simulink model "cirrusSR22T_v65"  (R2023a)
settings: Solver=ode45  StartTime=0.0  StopTime=360  FixedStep=0.001  MaxStep=0.1  RelTol=1e-3  EnableMultiTasking=on
values from neighbouring files (symbols this model uses):
  Aero_RP = [-1.145  0.0 -0.53]*[-1 0 0;0 1 0;0 0 -1]    [sr22t_data.m]
  aileron_limits = [-0.35 0.35]    [sr22t_data.m]
  Bw = 25.99*0.3048    (= 7.921752)    [sr22t_data.m]
  CD_alpha = [-1.57    1.500 ... (first row only)    [sr22t_data.m]
  CD_beta = [-1.57    1.230 ... (first row only)    [sr22t_data.m]
  CD_elev = 0.01    [sr22t_data.m]
  CD_ind = 0.007    [sr22t_data.m]
  CD_mach = [0, 0 ... (first row only)    [sr22t_data.m]
  Cl_ail = 0.1    [sr22t_data.m]
  CL_alpha = [-0.20 -0.750 ... (first row only)    [sr22t_data.m]
  Cl_beta = -0.1    [sr22t_data.m]
  CL_elev = 0.15    [sr22t_data.m]
  Cl_p = -0.4    [sr22t_data.m]
  CL_q = 3.9 * 0    (= 0)    [sr22t_data.m]
  Cl_r = 0.15    [sr22t_data.m]
  Cl_rudder = 0.01    [sr22t_data.m]
  Cm_alpha = -0.8    [sr22t_data.m]
  Cm_alpha_dot = -7    [sr22t_data.m]
  Cm_elev = [0.0, -1.100 ... (first row only)    [sr22t_data.m]
  Cm_q = -15    [sr22t_data.m]
  Cn_ail = -0.01    [sr22t_data.m]
  Cn_beta = 0.12    [sr22t_data.m]
  Cn_r = -0.15    [sr22t_data.m]
  Cn_rudder = -0.15    [sr22t_data.m]
  Cw = 5.58*0.3048    (= 1.700784)    [sr22t_data.m]
  CY_beta = -1    [sr22t_data.m]
  CY_p = [0.0000  -0.075 ... (first row only)    [sr22t_data.m]
  CY_r = [0.0000   0.214 ... (first row only)    [sr22t_data.m]
  CY_rudder = 0.187    [sr22t_data.m]
  Den = tf_linsys1(3,2).Denominator{1,1}    [controller_h_hold.m]
  elevator_limits = [-0.35 0.35]    [sr22t_data.m]
  He = tf_linsys1(3,2).Numerator{1,1}    [controller_h_hold.m]
  Href = 0.05 * x0(3)    [controller_h_hold.m]
  Ht = tf_linsys1(3,4).Numerator{1,1}    [controller_h_hold.m]
  isTrimming = 0    [sr22t_data.m]
  Jxx = 897*1.3558179    (= 1216.1686563)    [sr22t_data.m]
  Jxz = 0    [sr22t_data.m]
  Jyy = 20699*1.3558179    (= 28064.0747121)    [sr22t_data.m]
  Jzz = 19876*1.3558179    (= 26948.2365804)    [sr22t_data.m]
  Kp = 6    [controller_h_hold.m]
  kp = 0.005    [controller_h_hold.m]
  Kq = 3    [controller_h_hold.m]
  M = 2348*0.45359237    (= 1065.03488476)    [sr22t_data.m]
  Qe = tf_linsys1(8,2).Numerator{1,1}    [controller_h_hold.m]
  Qt = tf_linsys1(8,4).Numerator{1,1}    [controller_h_hold.m]
  Rcg = [-1.25 0.00 -0.54]*[-1 0 0;0 1 0;0 0 -1]    [sr22t_data.m]
  Rengine = [-3.6 0.0 -0.09045]*[-1 0 0;0 1 0;0 0 -1]    [sr22t_data.m]
  rudder_limits = [-0.35 0.35]    [sr22t_data.m]
  Sw = 144.92*0.09290304    (= 13.4635085568)    [sr22t_data.m]
  tau = 30    [controller_h_hold.m]
  Thetae = tf_linsys1(11,2).Numerator{1,1}    [controller_h_hold.m]
  Thetat = tf_linsys1(11,4).Numerator{1,1}    [controller_h_hold.m]
  thrust_limits = [0 1]    [sr22t_data.m]
  Ti = 17.5    [controller_h_hold.m]
  Tmax = M*10    (= 10650.3488476)    [sr22t_data.m]
  u0 = [op_trim1.Inputs(1,1).u, op_trim1.Inputs(2,1).u, op_trim1.Inputs(3,1).u, op_trim1.Inputs(4,1).u].'    [controller_h_hold.m]    (also in sr22t_data.m = [0, -0.013822, 0, 0.11837].')
  Ue = tf_linsys1(4,2).Numerator{1,1}    [controller_h_hold.m]
  Ut = tf_linsys1(4,4).Numerator{1,1}    [controller_h_hold.m]
  We = tf_linsys1(6,2).Numerator{1,1}    [controller_h_hold.m]
  Wt = tf_linsys1(6,4).Numerator{1,1}    [controller_h_hold.m]
  x0 = zeros(12,1)    [controller_h_hold.m]    (also in sr22t_data.m)
(part 1 of 2)
settings Model: Creator=torres  LastModifiedBy=santi
settings SolverCC: AlgebraicLoopSolver=TrustRegion
settings DataIOCC: LimitDataPoints=on  SaveFormat=Array  SignalLoggingSaveFormat=ModelDataLogs  SaveOutput=off  SaveTime=off  ReturnWorkspaceOutputs=off  SignalLoggingName=sigsOut
settings OptimizationCC: InitFltsAndDblsToZero=on  LifeSpan=inf
settings DebuggingCC: SaveWithParameterizedLinksMsg=none  UnderspecifiedInitializationDetection=Classic  MergeDetectMultiDrivingBlocksExec=none  SignalResolutionControl=TryResolveAllWithWarning  MultiTaskDSMMsg=warning  MultiTaskCondExecSysMsg=none  FcnCallInpInsideContextMsg=warning  UnconnectedInputMsg=warning  UnconnectedOutputMsg=warning  UnconnectedLineMsg=warning  SFUnexpectedBacktrackingDiag=warning  SFNoUnconditionalDefaultTransitionDiag=warning  SFExecutionAtInitializationDiag=none  ArithmeticOperatorsInVariantConditions=warning
settings HardwareCC: ProdBitPerPointer=32  ProdBitPerSizeT=32  ProdBitPerPtrDiffT=32  ProdLargestAtomicFloat=None  ProdIntDivRoundTo=Undefined  ProdEndianess=Unspecified  ProdWordSize=32  ProdHWDeviceType=32-bit Generic  TargetHWDeviceType=32-bit Generic  TargetUnknown=on  ProdEqTarget=off
settings ModelReferenceCC: PropagateSignalLabelsOutOfModel=off
settings CodeAppCC: StateflowObjectComments=on
settings GRTTargetCC: TargetFcnLib=ansi_tfl_tmw.mat  TargetLangStandard=C89/C90 (ANSI)  CombineOutputUpdateFcns=off  GRTInterface=on
settings ConfigComp: CovMetricSettings=dw  CovSaveCumulativeToWorkspaceVar=on  CovSaveSingleToWorkspaceVar=on

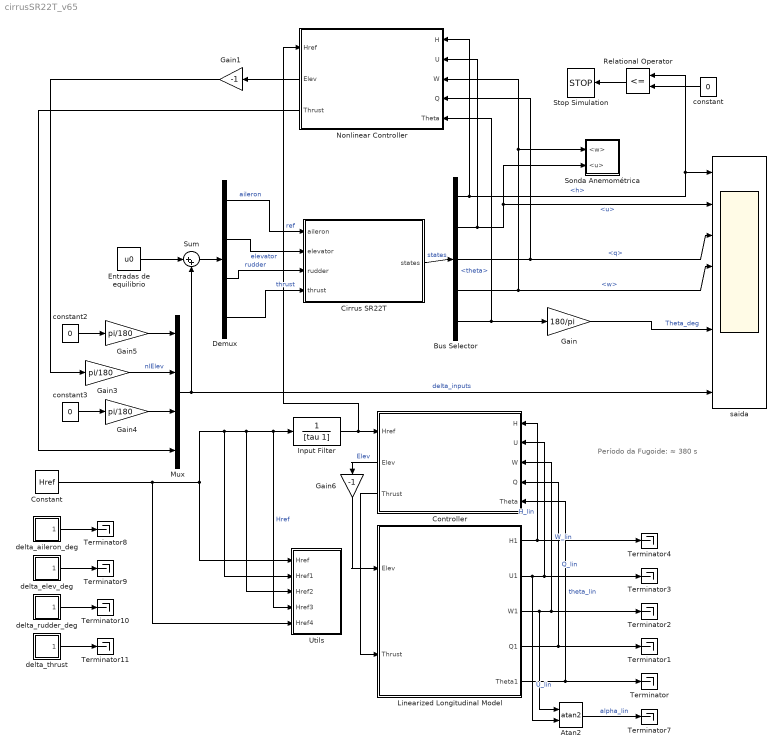
== system cirrusSR22T_v65 ==
  note: Período da Fugoide:
      | ≈ 380 s
  Atan2 : Trigonometry  Operator=atan2
  Bus Selector : BusSelector  OutputSignals=h,u,q,w,theta
  Cirrus SR22T : Subsystem
      mask Display: image(imread('SR22T.png'))
  Constant : Constant  Value=Href
  Controller : Subsystem
      settings: PortSchema="{\"entries\":[{\"content\":{\"sides\":[{\"content\":{\"connectorIds\":[\"In1\",\"In2\",\"In3\",\"In4\",\"In5\"]},\"type\":\"ConnectorPlacement.EquallySpacedRectSide\",\"uuid\":\"9a383977-e38d-4d96-a3fa-0666e6dce92b\"},{\"content\":{\"connectorIds\":[\"In6\",\"Out1\",\"Out2\"],\"side\":\"RIGHT\"},\"type\":\"ConnectorPlacement.EquallySpacedRectSide\",\"uuid\":\"65d7c93f-963c-4d71-9e25-46c931ae3c13\"},{\"content\":{\"side\":\"TOP\"},\"type\":\"ConnectorPlacement.EquallySpacedRectSide\",\"uuid\":\"543da9eb-7754-41f0-af2e-6eb03e83efa0\"}]},\"type\":\"ConnectorPlacement.EquallySpacedConnector\",\"uuid\":\"2a52e937-2907-406d-a0c6-1b75b66257ee\"}],\"packageUris\":[\"http://schema.mathworks.com/mf0/Connector/R2020b\"],\"version\":\"1.0\"}"
  Demux : Demux
      settings: DisplayOption=none
  Entradas de equilibrio : Constant  Value=u0
  Gain : Gain  Gain=180/pi  SaturateOnIntegerOverflow=on  OutDataTypeStr=Inherit: Same as input  ParamDataTypeStr=Inherit: Same as input
  Gain1 : Gain  Gain=-1
  Gain3 : Gain  Gain=pi/180  SaturateOnIntegerOverflow=on  OutDataTypeStr=Inherit: Same as input  ParamDataTypeStr=Inherit: Same as input
  Gain4 : Gain  Gain=pi/180  SaturateOnIntegerOverflow=on  OutDataTypeStr=Inherit: Same as input  ParamDataTypeStr=Inherit: Same as input
  Gain5 : Gain  Gain=pi/180  SaturateOnIntegerOverflow=on  OutDataTypeStr=Inherit: Same as input  ParamDataTypeStr=Inherit: Same as input
  Gain6 : Gain  Gain=-1
  Input Filter : TransferFcn  Denominator=[tau 1]
  Linearized Longitudinal Model : Subsystem
  Mux : Mux
  Nonlinear Controller : Subsystem
      settings: PortSchema="{\"entries\":[{\"content\":{\"sides\":[{\"content\":{\"connectorIds\":[\"In1\",\"In2\",\"In3\",\"In4\",\"In5\"]},\"type\":\"ConnectorPlacement.EquallySpacedRectSide\",\"uuid\":\"9a383977-e38d-4d96-a3fa-0666e6dce92b\"},{\"content\":{\"connectorIds\":[\"In6\",\"Out1\",\"Out2\"],\"side\":\"RIGHT\"},\"type\":\"ConnectorPlacement.EquallySpacedRectSide\",\"uuid\":\"65d7c93f-963c-4d71-9e25-46c931ae3c13\"},{\"content\":{\"side\":\"TOP\"},\"type\":\"ConnectorPlacement.EquallySpacedRectSide\",\"uuid\":\"543da9eb-7754-41f0-af2e-6eb03e83efa0\"}]},\"type\":\"ConnectorPlacement.EquallySpacedConnector\",\"uuid\":\"2a52e937-2907-406d-a0c6-1b75b66257ee\"}],\"packageUris\":[\"http://schema.mathworks.com/mf0/Connector/R2020b\"],\"version\":\"1.0\"}"
  Relational Operator : RelationalOperator  Operator=<=  InputSameDT=off
  Sonda Anemométrica : Subsystem
  Stop Simulation : Stop
  Sum : Sum  Inputs=|++  SaturateOnIntegerOverflow=on
  Terminator{,1..4,7..11} (10 alike) : Terminator
  Utils : Subsystem
  constant : Constant  Value=0
  constant2 : Constant  Value=0
  constant3 : Constant  Value=0
  delta_aileron_deg : Subsystem  mask{t0=90, dt=5, A=0}
      mask prompts: t0 "Start time"; dt "Pulse Width"; A "Amplitude"
      mask help: Doublet input to control surface.
      mask Display: plot(0,0,100,100,[90,70,70,50,50,30,30,10],[50,50,10,10,90,90,50,50])
  delta_elev_deg : Subsystem  mask{t0=20, dt=1, A=1}
      mask prompts: t0 "Start time"; dt "Pulse Width"; A "Amplitude"
      mask help: Doublet input to control surface.
      mask Display: plot(0,0,100,100,[90,70,70,50,50,30,30,10],[50,50,10,10,90,90,50,50])
  delta_rudder_deg : Subsystem  mask{t0=90, dt=1, A=0}
      mask prompts: t0 "Start time"; dt "Pulse Width"; A "Amplitude"
      mask help: Doublet input to control surface.
      mask Display: plot(0,0,100,100,[90,70,70,50,50,30,30,10],[50,50,10,10,90,90,50,50])
  delta_thrust : Subsystem  mask{t0=60, dt=1000, A=0}
      mask prompts: t0 "Start time"; dt "Duration"; A "Amplitude"
      mask Display: plot(0,0,100,100,[98,50,50,30,30,2],[20,20,80,80,20,20])
  saida : Scope  NumInputPorts=8
  wires:
  Cirrus SR22T/1(states) -> Bus Selector/1  "states"
  Bus Selector/2 -> Nonlinear Controller/2(U), saida/2, Sonda Anemométrica/2(<u>)  "<u>"
  Bus Selector/3 -> Nonlinear Controller/4(Q), saida/3  "<q>"
  Bus Selector/4 -> Nonlinear Controller/3(W), Sonda Anemométrica/1(<w>), saida/4  "<w>"
  Bus Selector/5 -> Gain/1, Nonlinear Controller/5(Theta)  "<theta>"
  Demux/1 -> Cirrus SR22T/1(aileron)  "aileron"
  Gain/1 -> saida/6  "Theta_deg"
  Demux/2 -> Cirrus SR22T/2(elevator)  "elevator"
  Demux/3 -> Cirrus SR22T/3(rudder)  "rudder"
  Demux/4 -> Cirrus SR22T/4(thrust)  "thrust"
  Entradas de equilibrio/1 -> Sum/1
  Sum/1 -> Demux/1
  constant2/1 -> Gain5/1
  Nonlinear Controller/1(Elev) -> Gain1/1
  constant3/1 -> Gain4/1
  Nonlinear Controller/2(Thrust) -> Mux/4
  Mux/1 -> Sum/2, saida/8  "delta_inputs"
  Gain3/1 -> Mux/2  "nlElev"
  Gain4/1 -> Mux/3
  Gain5/1 -> Mux/1
  Relational Operator/1 -> Stop Simulation/1
  constant/1 -> Relational Operator/2
  Bus Selector/1 -> Nonlinear Controller/1(H), Relational Operator/1, saida/1  "<h>"
  Linearized Longitudinal Model/5(Theta1) -> Controller/5(Theta), Terminator/1  "theta_lin"
  Linearized Longitudinal Model/4(Q1) -> Controller/4(Q), Terminator1/1  "Q_lin"
  Linearized Longitudinal Model/3(W1) -> Terminator2/1, Controller/3(W), Atan2/1  "W_lin"
  Linearized Longitudinal Model/2(U1) -> Terminator3/1, Controller/2(U), Atan2/2  "U_lin"
  Linearized Longitudinal Model/1(H1) -> Controller/1(H), Terminator4/1  "H_lin"
  Controller/2(Thrust) -> Linearized Longitudinal Model/2(Thrust)
  Controller/1(Elev) -> Gain6/1  "Elev"
  Gain6/1 -> Linearized Longitudinal Model/1(Elev)
  Atan2/1 -> Terminator7/1  "alpha_lin"
  delta_rudder_deg/1(Out1) -> Terminator10/1
  delta_elev_deg/1(Out1) -> Terminator9/1
  delta_aileron_deg/1(Out1) -> Terminator8/1
  delta_thrust/1(Out1) -> Terminator11/1
  Gain1/1 -> Gain3/1
  Constant/1 -> Utils/5(Href4), Utils/2(Href1), Utils/3(Href2), Utils/4(Href3), Input Filter/1, Utils/1(Href)  "Href"
  Input Filter/1 -> Nonlinear Controller/6(Href), Controller/6(Href)  "ref"

== system cirrusSR22T_v65/Cirrus SR22T ==
  note: Modelo Dinamico de Corpo Rigido
  aileron : Inport
  elevator : Inport  Port=2
  rudder : Inport  Port=3
  thrust : Inport  Port=4
  Aerodinamica : Subsystem  mask{flap=0, bw=Bw, cw=Cw, Sw=Sw}
      mask prompts: flap "Comando Flap (0, 1, 2 ou 3)"; bw "Comprimento da asa  - wingspan (m)"; cw "Corda media da asa (m)"; Sw "Area da asa (m2)"
  Atmosfera Padrao : Subsystem
  Bus Creator : BusCreator  Inputs=4
  Equations of Motion : Subsystem  mask{R_engine=Rengine, Rcg=Rcg, Aero_RP=Aero_RP, m=M, Jxz=Jxz, Jxx=Jxx, Jyy=Jyy, Jzz=Jzz, d=[0; 0; 0]}
      mask prompts: R_engine "Engine position (row vector in meters)"; Rcg "C.G. position (m)"; Aero_RP "Nominal C.G. (m) = Aerodynamic Reference Point"; m "Aircraft mass (Kg)"; Jxz "Inertia product (Jxz)"; Jxx "Inertia (Jxx)"; Jyy "Inertia (Jyy)"; Jzz "Inertia (Jzz)"; d "Accelerometers displacement from CG (vector in the ABC frame, in (m))"
  Gravidade : Constant  Value=9.807
  Propulsao : Subsystem  mask{Tmax=Tmax}
      mask prompts: Tmax "Tracao Maxima (N)"
  Saturation : Saturate  UpperLimit=aileron_limits(2)  LowerLimit=aileron_limits(1)
  Saturation1 : Saturate  UpperLimit=elevator_limits(2)  LowerLimit=elevator_limits(1)
  Saturation2 : Saturate  UpperLimit=rudder_limits(2)  LowerLimit=rudder_limits(1)
  Saturation3 : Saturate  UpperLimit=thrust_limits(2)  LowerLimit=thrust_limits(1)
  Terminator : Terminator
  Terminator1 : Terminator
  Terminator2 : Terminator
  states : Outport
  wires:
  Atmosfera Padrao/1(Atmosphere) -> Aerodinamica/3(Atmosphere)
  Equations of Motion/1(states) -> states/1, Aerodinamica/1(states), Atmosfera Padrao/1(states)
  aileron/1 -> Saturation/1  "aileron"
  elevator/1 -> Saturation1/1  "elevator"
  rudder/1 -> Saturation2/1  "rudder"
  Gravidade/1 -> Atmosfera Padrao/2(gravity), Equations of Motion/3(gravity)
  thrust/1 -> Saturation3/1  "thrust"
  Bus Creator/1 -> Aerodinamica/2(controls), Propulsao/1(controls)
  Aerodinamica/1(Faero) -> Equations of Motion/1(Faero)
  Aerodinamica/2(Maero) -> Equations of Motion/2(Maero)
  Propulsao/1(Thrust) -> Equations of Motion/4(Thrust)
  Saturation/1 -> Bus Creator/1  "aileron"
  Saturation1/1 -> Bus Creator/2  "elevator"
  Saturation2/1 -> Bus Creator/3  "rudder"
  Saturation3/1 -> Bus Creator/4  "thrust"
  Equations of Motion/2(ideal_gyro) -> Terminator/1
  Equations of Motion/4(ideal_attitude) -> Terminator2/1
  Equations of Motion/3(ideal_accelerometer) -> Terminator1/1

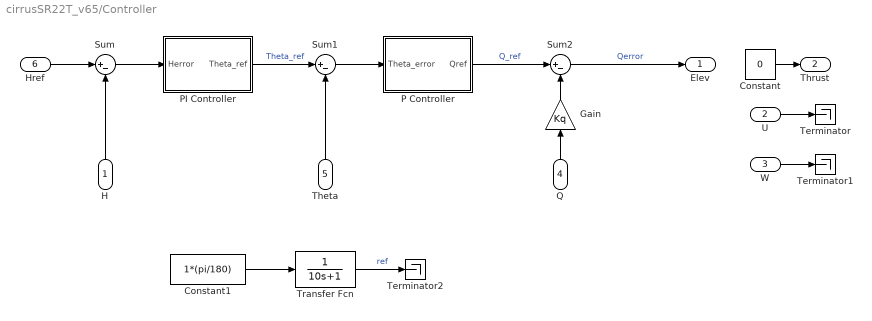
== system cirrusSR22T_v65/Controller ==
  H : Inport
  U : Inport  Port=2
  W : Inport  Port=3
  Q : Inport  Port=4
  Theta : Inport  Port=5
  Href : Inport  Port=6
  Constant : Constant  Value=0
  Constant1 : Constant  Value=1*(pi/180)  VectorParams1D=off
  Gain : Gain  Gain=Kq
  P Controller : Subsystem
  PI Controller : Subsystem
  Sum : Sum  Inputs=|+-
  Sum1 : Sum  Inputs=|+-
  Sum2 : Sum  Inputs=|+-
  Terminator : Terminator
  Terminator1 : Terminator
  Terminator2 : Terminator
  Transfer Fcn : TransferFcn  Denominator=[10 1]
  Elev : Outport
  Thrust : Outport  Port=2
  wires:
  Href/1 -> Sum/1
  Sum/1 -> PI Controller/1(Herror)
  Sum1/1 -> P Controller/1(Theta_error)
  Sum2/1 -> Elev/1  "Qerror"
  U/1 -> Terminator/1
  W/1 -> Terminator1/1
  Constant/1 -> Thrust/1
  H/1 -> Sum/2
  Theta/1 -> Sum1/2
  Q/1 -> Gain/1
  Gain/1 -> Sum2/2
  P Controller/1(Qref) -> Sum2/1  "Q_ref"
  Transfer Fcn/1 -> Terminator2/1  "ref"
  Constant1/1 -> Transfer Fcn/1
  PI Controller/1(Theta_ref) -> Sum1/1  "Theta_ref"

== system cirrusSR22T_v65/Linearized Longitudinal Model ==
  Elev : Inport
  Thrust : Inport  Port=2
  H : Subsystem
  Q : Subsystem
  Theta : Subsystem
  U : Subsystem
  W : Subsystem
  H1 : Outport
  U1 : Outport  Port=2
  W1 : Outport  Port=3
  Q1 : Outport  Port=4
  Theta1 : Outport  Port=5
  wires:
  U/1(U) -> U1/1
  Q/1(Q) -> Q1/1
  Elev/1 -> Theta/1(Elev), Q/1(Elev), W/1(Elev), U/1(Elev), H/1(Elev)
  H/1(H) -> H1/1
  Theta/1(Theta) -> Theta1/1
  Thrust/1 -> Q/2(Thrust), Theta/2(Thrust), W/2(Thrust), U/2(Thrust), H/2(Thrust)
  W/1(W) -> W1/1

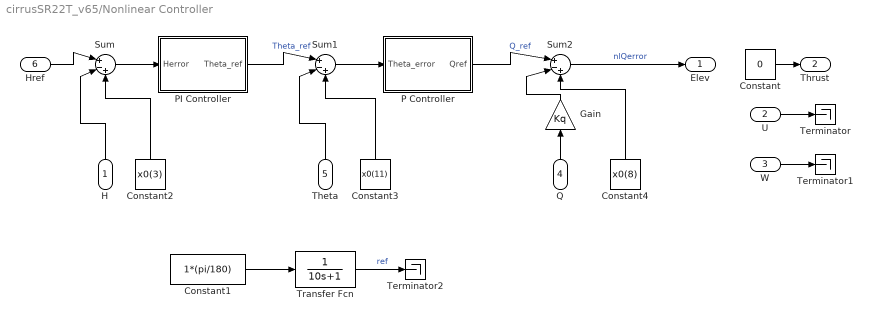
== system cirrusSR22T_v65/Nonlinear Controller ==
  H : Inport
  U : Inport  Port=2
  W : Inport  Port=3
  Q : Inport  Port=4
  Theta : Inport  Port=5
  Href : Inport  Port=6
  Constant : Constant  Value=0
  Constant1 : Constant  Value=1*(pi/180)  VectorParams1D=off
  Constant2 : Constant  Value=x0(3)
  Constant3 : Constant  Value=x0(11)
  Constant4 : Constant  Value=x0(8)
  Gain : Gain  Gain=Kq
  P Controller : Subsystem
  PI Controller : Subsystem
  Sum : Sum  Inputs=|+-+
  Sum1 : Sum  Inputs=|+-+
  Sum2 : Sum  Inputs=|+-+
  Terminator : Terminator
  Terminator1 : Terminator
  Terminator2 : Terminator
  Transfer Fcn : TransferFcn  Denominator=[10 1]
  Elev : Outport
  Thrust : Outport  Port=2
  wires:
  Href/1 -> Sum/1
  Sum/1 -> PI Controller/1(Herror)
  Sum1/1 -> P Controller/1(Theta_error)
  Sum2/1 -> Elev/1  "nlQerror"
  U/1 -> Terminator/1
  W/1 -> Terminator1/1
  Constant/1 -> Thrust/1
  H/1 -> Sum/2
  Theta/1 -> Sum1/2
  Q/1 -> Gain/1
  Gain/1 -> Sum2/2
  P Controller/1(Qref) -> Sum2/1  "Q_ref"
  Transfer Fcn/1 -> Terminator2/1  "ref"
  Constant1/1 -> Transfer Fcn/1
  PI Controller/1(Theta_ref) -> Sum1/1  "Theta_ref"
  Constant2/1 -> Sum/3
  Constant3/1 -> Sum1/3
  Constant4/1 -> Sum2/3

== system cirrusSR22T_v65/Sonda Anemométrica ==
  <w> : Inport
  <u> : Inport  Port=2
  Bus Selector3 : BusSelector  OutputSignals=VT,alpha,beta
  Gain7 : Gain  Gain=180/pi  SaturateOnIntegerOverflow=on  OutDataTypeStr=Inherit: Same as input  ParamDataTypeStr=Inherit: Same as input
  Gain8 : Gain  Gain=180/pi  SaturateOnIntegerOverflow=on  OutDataTypeStr=Inherit: Same as input  ParamDataTypeStr=Inherit: Same as input
  Mux1 : Mux  Inputs=3
  Sonda__anemometrica : Scope  NumInputPorts=3
  constant1 : Constant  Value=0
  "u,v,w -> Vt,alpha,beta" : Subsystem
  wires:
  Bus Selector3/1 -> Sonda__anemometrica/1  "<VT>"
  Gain7/1 -> Sonda__anemometrica/2  "alfa_deg"
  "u,v,w -> Vt,alpha,beta"/1(vel_wind) -> Bus Selector3/1
  Mux1/1 -> "u,v,w -> Vt,alpha,beta"/1(vel_body)
  constant1/1 -> Mux1/2
  Bus Selector3/3 -> Gain8/1  "<beta>"
  Gain8/1 -> Sonda__anemometrica/3  "beta_deg"
  Bus Selector3/2 -> Gain7/1  "<alpha>"
  <w>/1 -> Mux1/3
  <u>/1 -> Mux1/1

== system cirrusSR22T_v65/Utils ==
  Href : Inport
  Href1 : Inport  Port=2
  Href2 : Inport  Port=3
  Href3 : Inport  Port=4
  Href4 : Inport  Port=5
  Constant1 : Constant  Value=x0(3)
  Gain10 : Gain  Gain=-0.02
  Gain9 : Gain  Gain=0.02
  Sum{1..5} (5 alike) : Sum  Inputs=|++
  Terminator12 : Terminator
  Terminator5 : Terminator
  Terminator6 : Terminator
  wires:
  Sum3/1 -> Terminator5/1  "nlHref+"
  Sum5/1 -> Terminator12/1  "nlHref"
  Gain10/1 -> Sum2/1
  Href/1 -> Gain9/1
  Constant1/1 -> Sum3/2, Sum5/2, Sum4/2
  Sum4/1 -> Terminator6/1  "nlHref-"
  Sum1/1 -> Sum3/1  "Href+"
  Gain9/1 -> Sum1/1
  Sum2/1 -> Sum4/1  "Href-"
  Href4/1 -> Sum5/1
  Href1/1 -> Sum1/2
  Href3/1 -> Sum2/2
  Href2/1 -> Gain10/1

== system cirrusSR22T_v65/delta_aileron_deg ==
  Step : Step  Time=t0  After=A  SampleTime=0
  Step1 : Step  Time=t0+dt  After=-2*A  SampleTime=0
  Step2 : Step  Time=t0+2*dt  After=A  SampleTime=0
  Sum : Sum  Inputs=|++  SaturateOnIntegerOverflow=on
  Sum1 : Sum  Inputs=|++  SaturateOnIntegerOverflow=on
  Out1 : Outport
  wires:
  Step/1 -> Sum/1
  Step1/1 -> Sum/2
  Sum/1 -> Sum1/1
  Sum1/1 -> Out1/1
  Step2/1 -> Sum1/2

== system cirrusSR22T_v65/delta_elev_deg ==
  Step : Step  Time=t0  After=A  SampleTime=0
  Step1 : Step  Time=t0+dt  After=-2*A  SampleTime=0
  Step2 : Step  Time=t0+2*dt  After=A  SampleTime=0
  Sum : Sum  Inputs=|++  SaturateOnIntegerOverflow=on
  Sum1 : Sum  Inputs=|++  SaturateOnIntegerOverflow=on
  Out1 : Outport
  wires:
  Step/1 -> Sum/1
  Step1/1 -> Sum/2
  Sum/1 -> Sum1/1
  Sum1/1 -> Out1/1
  Step2/1 -> Sum1/2

== system cirrusSR22T_v65/delta_rudder_deg ==
  Step : Step  Time=t0  After=A  SampleTime=0
  Step1 : Step  Time=t0+dt  After=-2*A  SampleTime=0
  Step2 : Step  Time=t0+2*dt  After=A  SampleTime=0
  Sum : Sum  Inputs=|++  SaturateOnIntegerOverflow=on
  Sum1 : Sum  Inputs=|++  SaturateOnIntegerOverflow=on
  Out1 : Outport
  wires:
  Step/1 -> Sum/1
  Step1/1 -> Sum/2
  Sum/1 -> Sum1/1
  Sum1/1 -> Out1/1
  Step2/1 -> Sum1/2

== system cirrusSR22T_v65/delta_thrust ==
  Step : Step  Time=t0  After=A  SampleTime=0
  Step1 : Step  Time=t0+dt  After=-A  SampleTime=0
  Sum : Sum  Inputs=|++  SaturateOnIntegerOverflow=on
  Out1 : Outport
  wires:
  Sum/1 -> Out1/1
  Step/1 -> Sum/1
  Step1/1 -> Sum/2

== system cirrusSR22T_v65/Cirrus SR22T/Aerodinamica ==
  states : Inport
  controls : Inport  Port=2
  Atmosphere : Inport  Port=3
  Bus Selector : BusSelector  OutputSignals=u,v,w,p,q,r
  Bus Selector2 : BusSelector  OutputSignals=aileron,elevator,rudder
  Bus Selector3 : BusSelector  OutputSignals=VT,alpha,beta
  Bus Selector4 : BusSelector  OutputSignals=VT,alpha,beta
  Calc_qbar_Mach : Subsystem
  Derivative : Derivative
  Forcas Aerodinamicas : Subsystem
  ForcasMomentos : Scope  NumInputPorts=2
  Momentos Aerodinamicos : Subsystem
  Mux : Mux  Inputs=3
  Wind->ABC : Subsystem
  "u,v,w -> Vt,alpha,beta" : Subsystem
  Faero : Outport
  Maero : Outport  Port=2
  wires:
  Bus Selector/4 -> Forcas Aerodinamicas/4(p), Momentos Aerodinamicos/5(p)  "<p>"
  Bus Selector2/2 -> Momentos Aerodinamicos/9(elevator), Forcas Aerodinamicas/8(elevator)  "<elevator>"
  Bus Selector/6 -> Forcas Aerodinamicas/6(r), Momentos Aerodinamicos/7(r)  "<r>"
  Bus Selector4/2 -> Momentos Aerodinamicos/2(alpha), Derivative/1  "<alpha>"
  Bus Selector3/2 -> Wind->ABC/1(alpha), Forcas Aerodinamicas/2(alpha)  "<alpha>"
  Bus Selector3/3 -> Wind->ABC/2(beta), Forcas Aerodinamicas/3(beta)  "<beta>"
  Bus Selector2/1 -> Momentos Aerodinamicos/10(aileron)  "<aileron>"
  controls/1 -> Bus Selector2/1
  Bus Selector3/1 -> Forcas Aerodinamicas/1(VT), Calc_qbar_Mach/2(<VT>)  "<VT>"
  Bus Selector4/3 -> Momentos Aerodinamicos/4(beta)  "<beta>"
  Atmosphere/1 -> Calc_qbar_Mach/1(In1)
  "u,v,w -> Vt,alpha,beta"/1(vel_wind) -> Bus Selector4/1, Bus Selector3/1
  states/1 -> Bus Selector/1
  Mux/1 -> "u,v,w -> Vt,alpha,beta"/1(vel_body)
  Forcas Aerodinamicas/1(Faero_wind) -> Wind->ABC/3(V_Wind), ForcasMomentos/1
  Bus Selector2/3 -> Momentos Aerodinamicos/8(rudder), Forcas Aerodinamicas/7(rudder)  "<rudder>"
  Bus Selector4/1 -> Momentos Aerodinamicos/1(VT)  "<VT>"
  Wind->ABC/1(V_ABC) -> Faero/1
  Bus Selector/1 -> Mux/1  "<u>"
  Calc_qbar_Mach/1(qbar) -> Momentos Aerodinamicos/11(pressao_dinamica_total), Momentos Aerodinamicos/12(pressao_dinamica), Forcas Aerodinamicas/9(pressao_dinamica)
  Bus Selector/3 -> Mux/3  "<w>"
  Derivative/1 -> Momentos Aerodinamicos/3(alpha_dot)
  Bus Selector/5 -> Forcas Aerodinamicas/5(q), Momentos Aerodinamicos/6(q)  "<q>"
  Calc_qbar_Mach/2(Mach) -> Forcas Aerodinamicas/10(Mach), Momentos Aerodinamicos/13(Mach)
  Bus Selector/2 -> Mux/2  "<v>"
  Momentos Aerodinamicos/1(Maero_body) -> ForcasMomentos/2, Maero/1

== system cirrusSR22T_v65/Cirrus SR22T/Atmosfera Padrao ==
  states : Inport
  gravity : Inport  Port=2
  Bus Creator : BusCreator  Inputs=4
  Bus Selector : BusSelector  OutputSignals=h
  Calc. Densidade : Fcn  Expr=1.225*(u(1)/288.15)^(-u(2)/(-0.0065*287.04)-1)
  Calc. Pressao : Fcn  Expr=101325*(u(1)/288.15)^(-u(2)/(-0.0065*287.04))
  Calc. Temperatura : Fcn  Expr=288.15 -0.0065*u(1)
  Calc. Vel. Som : Fcn  Expr=sqrt(u*1.4*287.04)
  Mux : Mux  Inputs=2
  Mux1 : Mux  Inputs=2
  Atmosphere : Outport
  wires:
  states/1 -> Bus Selector/1
  Bus Selector/1 -> Mux/1  "<h>"
  gravity/1 -> Mux/2, Mux1/2
  Mux/1 -> Calc. Temperatura/1
  Mux1/1 -> Calc. Pressao/1, Calc. Densidade/1
  Calc. Temperatura/1 -> Mux1/1, Calc. Vel. Som/1, Bus Creator/3  "Temperatura (K)"
  Calc. Pressao/1 -> Bus Creator/4  "Pressao (Pa)"
  Calc. Densidade/1 -> Bus Creator/1  "densidade (Kg/m3)"
  Calc. Vel. Som/1 -> Bus Creator/2  "Vel_som (m/s)"
  Bus Creator/1 -> Atmosphere/1

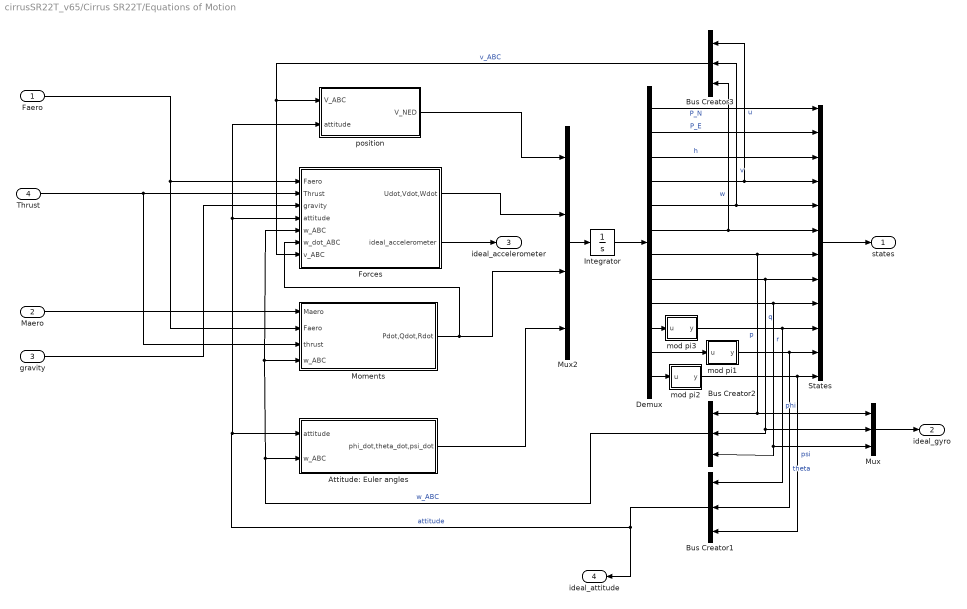
== system cirrusSR22T_v65/Cirrus SR22T/Equations of Motion ==
  Faero : Inport
  Maero : Inport  Port=2
  gravity : Inport  Port=3
  Thrust : Inport  Port=4
  Attitude: Euler angles : Subsystem
  Bus Creator1 : BusCreator  Inputs=3
  Bus Creator2 : BusCreator  Inputs=3
  Bus Creator3 : BusCreator  Inputs=3
  Demux : Demux  Outputs=12
      settings: DisplayOption=none
  Forces : Subsystem
  Integrator : Integrator  InitialCondition=x0
  Moments : Subsystem
  Mux : Mux  Inputs=3
  Mux2 : Mux
  States : BusCreator  Inputs=12
  mod pi1 : Subsystem
  mod pi2 : Subsystem
  mod pi3 : Subsystem
  position : Subsystem
  states : Outport
  ideal_gyro : Outport  Port=2
  ideal_accelerometer : Outport  Port=3
  ideal_attitude : Outport  Port=4
  wires:
  Demux/3 -> States/3  "h"
  Demux/4 -> States/4, Bus Creator3/1  "u"
  Demux/5 -> States/5, Bus Creator3/2  "v"
  Demux/6 -> States/6, Bus Creator3/3  "w"
  Demux/7 -> States/7, Bus Creator2/1, Mux/1  "p"
  Demux/8 -> States/8, Bus Creator2/2, Mux/2  "q"
  Demux/9 -> States/9, Bus Creator2/3, Mux/3  "r"
  Demux/10 -> mod pi3/1(u)
  Demux/11 -> mod pi1/1(u)
  Demux/12 -> mod pi2/1(u)
  Integrator/1 -> Demux/1
  States/1 -> states/1
  Mux2/1 -> Integrator/1
  Thrust/1 -> Moments/3(thrust), Forces/2(Thrust)
  Bus Creator1/1 -> Attitude: Euler angles/1(attitude), Forces/4(attitude), position/2(attitude), ideal_attitude/1  "attitude"
  Forces/1(Udot,Vdot,Wdot) -> Mux2/2
  gravity/1 -> Forces/3(gravity)
  Attitude: Euler angles/1(phi_dot,theta_dot,psi_dot) -> Mux2/4
  Maero/1 -> Moments/1(Maero)
  Bus Creator3/1 -> Forces/7(v_ABC), position/1(V_ABC)  "v_ABC"
  Faero/1 -> Forces/1(Faero), Moments/2(Faero)
  Bus Creator2/1 -> Attitude: Euler angles/2(w_ABC), Forces/5(w_ABC), Moments/4(w_ABC)  "w_ABC"
  Moments/1(Pdot,Qdot,Rdot) -> Mux2/3, Forces/6(w_dot_ABC)
  Demux/1 -> States/1  "P_N"
  Demux/2 -> States/2  "P_E"
  position/1(V_NED) -> Mux2/1
  mod pi3/1(y) -> States/10, Bus Creator1/1  "phi"
  mod pi1/1(y) -> States/11, Bus Creator1/2  "theta"
  mod pi2/1(y) -> States/12, Bus Creator1/3  "psi"
  Mux/1 -> ideal_gyro/1
  Forces/2(ideal_accelerometer) -> ideal_accelerometer/1

== system cirrusSR22T_v65/Cirrus SR22T/Propulsao ==
  controls : Inport
  Bus Selector : BusSelector  OutputSignals=thrust
  Constant : Constant  Value=0
  Gain : Gain  Gain=Tmax  SaturateOnIntegerOverflow=on  OutDataTypeStr=Inherit: Same as input  ParamDataTypeStr=Inherit: Same as input
  Mux : Mux  Inputs=3
  Saturation : Saturate  UpperLimit=1  LowerLimit=0.0
  Thrust : Outport
  wires:
  Saturation/1 -> Gain/1
  controls/1 -> Bus Selector/1
  Bus Selector/1 -> Saturation/1  "<thrust>"
  Gain/1 -> Mux/1
  Mux/1 -> Thrust/1
  Constant/1 -> Mux/3, Mux/2

== system cirrusSR22T_v65/Controller/P Controller ==
  Theta_error : Inport
  Gain : Gain  Gain=Kp
  Qref : Outport
  wires:
  Theta_error/1 -> Gain/1  "Theta_error"
  Gain/1 -> Qref/1

== system cirrusSR22T_v65/Controller/PI Controller ==
  Herror : Inport
  Gain : Gain  Gain=kp
  Gain1 : Gain  Gain=1/Ti
  Integrator : Integrator
  Sum : Sum  Inputs=|++
  Theta_ref : Outport
  wires:
  Gain/1 -> Gain1/1, Sum/1
  Sum/1 -> Theta_ref/1
  Gain1/1 -> Integrator/1
  Herror/1 -> Gain/1  "Herror"
  Integrator/1 -> Sum/2

== system cirrusSR22T_v65/Linearized Longitudinal Model/H ==
  Elev : Inport
  Thrust : Inport  Port=2
  Sum1 : Sum  Inputs=|++
  Transfer Fcn : TransferFcn  Numerator=He  Denominator=Den
  Transfer Fcn1 : TransferFcn  Numerator=Ht  Denominator=Den
  H : Outport
  wires:
  Transfer Fcn/1 -> Sum1/1
  Elev/1 -> Transfer Fcn/1
  Sum1/1 -> H/1
  Transfer Fcn1/1 -> Sum1/2
  Thrust/1 -> Transfer Fcn1/1

== system cirrusSR22T_v65/Linearized Longitudinal Model/Q ==
  Elev : Inport
  Thrust : Inport  Port=2
  Sum1 : Sum  Inputs=|++
  Transfer Fcn : TransferFcn  Numerator=Qe  Denominator=Den
  Transfer Fcn1 : TransferFcn  Numerator=Qt  Denominator=Den
  Q : Outport
  wires:
  Transfer Fcn/1 -> Sum1/1
  Elev/1 -> Transfer Fcn/1
  Sum1/1 -> Q/1
  Transfer Fcn1/1 -> Sum1/2
  Thrust/1 -> Transfer Fcn1/1

== system cirrusSR22T_v65/Linearized Longitudinal Model/Theta ==
  Elev : Inport
  Thrust : Inport  Port=2
  Sum1 : Sum  Inputs=|++
  Transfer Fcn : TransferFcn  Numerator=Thetae  Denominator=Den
  Transfer Fcn1 : TransferFcn  Numerator=Thetat  Denominator=Den
  Theta : Outport
  wires:
  Transfer Fcn/1 -> Sum1/1
  Elev/1 -> Transfer Fcn/1
  Sum1/1 -> Theta/1
  Transfer Fcn1/1 -> Sum1/2
  Thrust/1 -> Transfer Fcn1/1

== system cirrusSR22T_v65/Linearized Longitudinal Model/U ==
  Elev : Inport
  Thrust : Inport  Port=2
  Sum1 : Sum  Inputs=|++
  Transfer Fcn : TransferFcn  Numerator=Ue  Denominator=Den
  Transfer Fcn1 : TransferFcn  Numerator=Ut  Denominator=Den
  U : Outport
  wires:
  Transfer Fcn/1 -> Sum1/1
  Elev/1 -> Transfer Fcn/1
  Sum1/1 -> U/1
  Transfer Fcn1/1 -> Sum1/2
  Thrust/1 -> Transfer Fcn1/1

== system cirrusSR22T_v65/Linearized Longitudinal Model/W ==
  Elev : Inport
  Thrust : Inport  Port=2
  Sum1 : Sum  Inputs=|++
  Transfer Fcn : TransferFcn  Numerator=We  Denominator=Den
  Transfer Fcn1 : TransferFcn  Numerator=Wt  Denominator=Den
  W : Outport
  wires:
  Transfer Fcn/1 -> Sum1/1
  Elev/1 -> Transfer Fcn/1
  Sum1/1 -> W/1
  Transfer Fcn1/1 -> Sum1/2
  Thrust/1 -> Transfer Fcn1/1

== system cirrusSR22T_v65/Nonlinear Controller/P Controller ==
  Theta_error : Inport
  Gain : Gain  Gain=Kp
  Qref : Outport
  wires:
  Theta_error/1 -> Gain/1  "nlTheta_error"
  Gain/1 -> Qref/1

== system cirrusSR22T_v65/Nonlinear Controller/PI Controller ==
  Herror : Inport
  Gain : Gain  Gain=kp
  Gain1 : Gain  Gain=1/Ti
  Integrator : Integrator
  Sum : Sum  Inputs=|++
  Theta_ref : Outport
  wires:
  Herror/1 -> Gain/1  "nlHerror"
  Gain1/1 -> Integrator/1
  Sum/1 -> Theta_ref/1
  Gain/1 -> Gain1/1, Sum/1
  Integrator/1 -> Sum/2

== system cirrusSR22T_v65/Sonda Anemométrica/u,v,w -> Vt,alpha,beta ==
  vel_body : Inport
  Bus Creator : BusCreator  Inputs=3
  VT : Fcn  Expr=sqrt(u(1)^2+u(2)^2+u(3)^2)
  alpha : Fcn  Expr=atan2(u(3),u(1))
  beta : Fcn  Expr=atan2(u(2),sqrt(u(1)^2+u(3)^2))
  vel_wind : Outport
  wires:
  Bus Creator/1 -> vel_wind/1
  VT/1 -> Bus Creator/1  "VT"
  alpha/1 -> Bus Creator/2  "alpha"
  vel_body/1 -> alpha/1, VT/1, beta/1
  beta/1 -> Bus Creator/3  "beta"

== system cirrusSR22T_v65/Cirrus SR22T/Aerodinamica/Calc_qbar_Mach ==
  In1 : Inport
  <VT> : Inport  Port=2
  Bus Selector1 : BusSelector  OutputSignals=densidade (Kg/m3),Vel_som (m/s)
  Gain : Gain  Gain=0.5
  Product : Product
  Product1 : Product  Inputs=*/
  Square : Math  Operator=square
  qbar : Outport
  Mach : Outport  Port=2
  wires:
  In1/1 -> Bus Selector1/1
  Product1/1 -> Mach/1
  Gain/1 -> qbar/1
  Bus Selector1/2 -> Product1/2  "<Vel_som (m/s)>"
  Product/1 -> Gain/1
  Square/1 -> Product/1
  Bus Selector1/1 -> Product/2  "<densidade (Kg/m3)>"
  <VT>/1 -> Square/1, Product1/1

== system cirrusSR22T_v65/Cirrus SR22T/Aerodinamica/Forcas Aerodinamicas ==
  note: Valores negativos para D e L para que fiquem consistentes com os eixos do Vento, como definidos por nós no curso.
  VT : Inport
  alpha : Inport  Port=2
  beta : Inport  Port=3
  p : Inport  Port=4
  q : Inport  Port=5
  r : Inport  Port=6
  rudder : Inport  Port=7
  elevator : Inport  Port=8
  pressao_dinamica : Inport  Port=9
  Mach : Inport  Port=10
  Coef. Arrasto : Subsystem
  Coef. Forca Lateral : Subsystem
  Coef. sustentacao : Subsystem
  Gain : Gain  Gain=-1
  Gain1 : Gain  Gain=-1
  Gain3 : Gain  Gain=Sw  SaturateOnIntegerOverflow=on  OutDataTypeStr=Inherit: Same as input  ParamDataTypeStr=Inherit: Same as input
  Mux : Mux  Inputs=3
  Product1 : Product  SaturateOnIntegerOverflow=on  OutDataTypeStr=Inherit: Same as first input
  Faero_wind : Outport
  wires:
  Coef. Forca Lateral/1(C_Y) -> Mux/2
  alpha/1 -> Coef. Arrasto/1(alpha), Coef. sustentacao/1(alpha), Coef. Forca Lateral/1(alpha)
  beta/1 -> Coef. Forca Lateral/2(beta), Coef. Arrasto/2(beta)
  VT/1 -> Coef. Forca Lateral/4(VT), Coef. sustentacao/3(VT)
  p/1 -> Coef. Forca Lateral/3(p)
  q/1 -> Coef. sustentacao/4(q)
  r/1 -> Coef. Forca Lateral/5(r)
  rudder/1 -> Coef. Forca Lateral/6(rudder)
  elevator/1 -> Coef. sustentacao/2(elevator), Coef. Arrasto/3(elevator)
  Mux/1 -> Product1/1
  Product1/1 -> Gain3/1
  Gain3/1 -> Faero_wind/1
  pressao_dinamica/1 -> Product1/2
  Coef. Arrasto/1(C_D) -> Gain/1
  Coef. sustentacao/1(C_L) -> Gain1/1
  Gain/1 -> Mux/1
  Gain1/1 -> Mux/3, Coef. Arrasto/4(C_L)
  Mach/1 -> Coef. Arrasto/5(Mach)

== system cirrusSR22T_v65/Cirrus SR22T/Aerodinamica/Momentos Aerodinamicos ==
  VT : Inport
  alpha : Inport  Port=2
  alpha_dot : Inport  Port=3
  beta : Inport  Port=4
  p : Inport  Port=5
  q : Inport  Port=6
  r : Inport  Port=7
  rudder : Inport  Port=8
  elevator : Inport  Port=9
  aileron : Inport  Port=10
  pressao_dinamica_total : Inport  Port=11
  pressao_dinamica : Inport  Port=12
  Mach : Inport  Port=13
  Coef. arfagem x cw : Subsystem
  Coef. guinada x bw : Subsystem
  Coef. rolamento x bw : Subsystem
  Gain3 : Gain  Gain=Sw  SaturateOnIntegerOverflow=on  OutDataTypeStr=Inherit: Same as input  ParamDataTypeStr=Inherit: Same as input
  Mux : Mux  Inputs=3
  Pdyn : Scope
  Maero_body : Outport
  wires:
  alpha/1 -> Coef. arfagem x cw/1(alpha)
  beta/1 -> Coef. guinada x bw/1(beta), Coef. rolamento x bw/1(beta)
  VT/1 -> Coef. rolamento x bw/2(VT), Coef. guinada x bw/2(VT), Coef. arfagem x cw/3(VT)
  p/1 -> Coef. rolamento x bw/3(p)
  r/1 -> Coef. rolamento x bw/4(r), Coef. guinada x bw/3(r)
  alpha_dot/1 -> Coef. arfagem x cw/2(alpha_dot)
  q/1 -> Coef. arfagem x cw/4(q)
  rudder/1 -> Coef. rolamento x bw/6(rudder), Coef. guinada x bw/5(rudder)
  elevator/1 -> Coef. arfagem x cw/5(elevator)
  aileron/1 -> Coef. rolamento x bw/5(aileron), Coef. guinada x bw/4(aileron)
  Mux/1 -> Gain3/1
  Coef. rolamento x bw/1(Cl_bw) -> Mux/1
  Coef. guinada x bw/1(Cn_bw) -> Mux/3
  Gain3/1 -> Maero_body/1
  Coef. arfagem x cw/1(Cm_cw) -> Mux/2
  pressao_dinamica/1 -> Pdyn/1, Coef. guinada x bw/6(pressao_dinamica), Coef. rolamento x bw/7(pressao_dinamica), Coef. arfagem x cw/6(pressao_dinamica)
  pressao_dinamica_total/1 -> Coef. rolamento x bw/8(pressao_dinamica_total), Coef. arfagem x cw/7(pressao_dinamica_total), Coef. guinada x bw/7(pressao_dinamica_total)
  Mach/1 -> Coef. arfagem x cw/8(Mach)

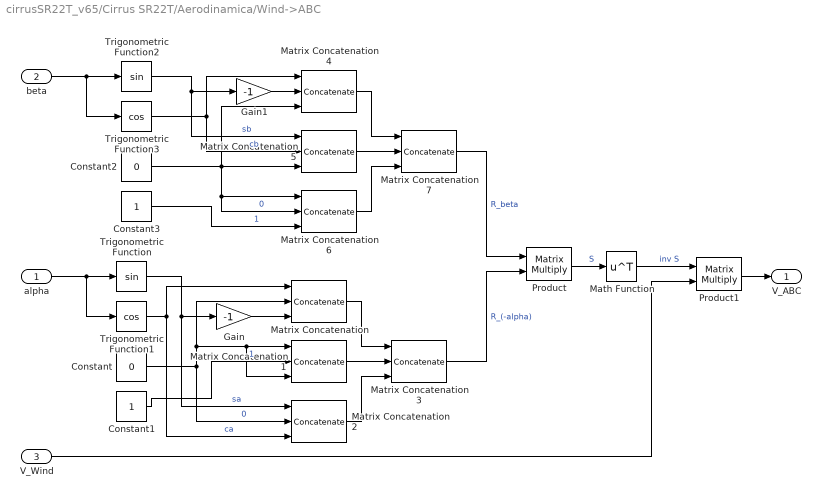
== system cirrusSR22T_v65/Cirrus SR22T/Aerodinamica/Wind->ABC ==
  alpha : Inport
  beta : Inport  Port=2
  V_Wind : Inport  Port=3
  Constant : Constant  Value=0
  Constant1 : Constant
  Constant2 : Constant  Value=0
  Constant3 : Constant
  Gain : Gain  Gain=-1  SaturateOnIntegerOverflow=on  OutDataTypeStr=Inherit: Same as input  ParamDataTypeStr=Inherit: Same as input
  Gain1 : Gain  Gain=-1  SaturateOnIntegerOverflow=on  OutDataTypeStr=Inherit: Same as input  ParamDataTypeStr=Inherit: Same as input
  Math Function : Math  Operator=transpose  SignedPower=on
  Matrix Concatenation{,1..2,4..6} (6 alike) : Concatenate  NumInputs=3  Mode=Multidimensional array
  Matrix Concatenation3 : Concatenate  NumInputs=3  Mode=Multidimensional array  ConcatenateDimension=2
  Matrix Concatenation7 : Concatenate  NumInputs=3  Mode=Multidimensional array  ConcatenateDimension=2
  Product : Product  Multiplication=Matrix(*)  SaturateOnIntegerOverflow=on  OutDataTypeStr=Inherit: Same as first input
  Product1 : Product  Multiplication=Matrix(*)  SaturateOnIntegerOverflow=on  OutDataTypeStr=Inherit: Same as first input
  Trigonometric Function : Trigonometry
  Trigonometric Function1 : Trigonometry  Operator=cos
  Trigonometric Function2 : Trigonometry
  Trigonometric Function3 : Trigonometry  Operator=cos
  V_ABC : Outport
  wires:
  alpha/1 -> Trigonometric Function/1, Trigonometric Function1/1
  Trigonometric Function1/1 -> Matrix Concatenation/1, Matrix Concatenation2/3  "ca"
  Trigonometric Function/1 -> Matrix Concatenation2/1, Gain/1  "sa"
  Constant/1 -> Matrix Concatenation/2, Matrix Concatenation1/1, Matrix Concatenation1/3, Matrix Concatenation2/2  "0"
  Constant1/1 -> Matrix Concatenation1/2  "1"
  Matrix Concatenation/1 -> Matrix Concatenation3/1
  Matrix Concatenation1/1 -> Matrix Concatenation3/2
  Matrix Concatenation2/1 -> Matrix Concatenation3/3
  Product/1 -> Math Function/1  "S"
  Math Function/1 -> Product1/1  "inv S"
  Product1/1 -> V_ABC/1
  beta/1 -> Trigonometric Function2/1, Trigonometric Function3/1
  Matrix Concatenation4/1 -> Matrix Concatenation7/1
  Matrix Concatenation5/1 -> Matrix Concatenation7/2
  Matrix Concatenation6/1 -> Matrix Concatenation7/3
  Trigonometric Function3/1 -> Matrix Concatenation4/1, Matrix Concatenation5/2  "cb"
  Trigonometric Function2/1 -> Gain1/1, Matrix Concatenation5/1  "sb"
  Constant2/1 -> Matrix Concatenation4/3, Matrix Concatenation5/3, Matrix Concatenation6/1, Matrix Concatenation6/2  "0"
  Constant3/1 -> Matrix Concatenation6/3  "1"
  Matrix Concatenation7/1 -> Product/1  "R_beta"
  Matrix Concatenation3/1 -> Product/2  "R_(-alpha)"
  Gain1/1 -> Matrix Concatenation4/2
  V_Wind/1 -> Product1/2
  Gain/1 -> Matrix Concatenation/3

== system cirrusSR22T_v65/Cirrus SR22T/Aerodinamica/u,v,w -> Vt,alpha,beta ==
  vel_body : Inport
  Bus Creator : BusCreator  Inputs=3
  VT : Fcn  Expr=sqrt(u(1)^2+u(2)^2+u(3)^2)
  alpha : Fcn  Expr=atan2(u(3),u(1))
  beta : Fcn  Expr=atan2(u(2),sqrt(u(1)^2+u(3)^2))
  vel_wind : Outport
  wires:
  Bus Creator/1 -> vel_wind/1
  VT/1 -> Bus Creator/1  "VT"
  alpha/1 -> Bus Creator/2  "alpha"
  vel_body/1 -> alpha/1, VT/1, beta/1
  beta/1 -> Bus Creator/3  "beta"

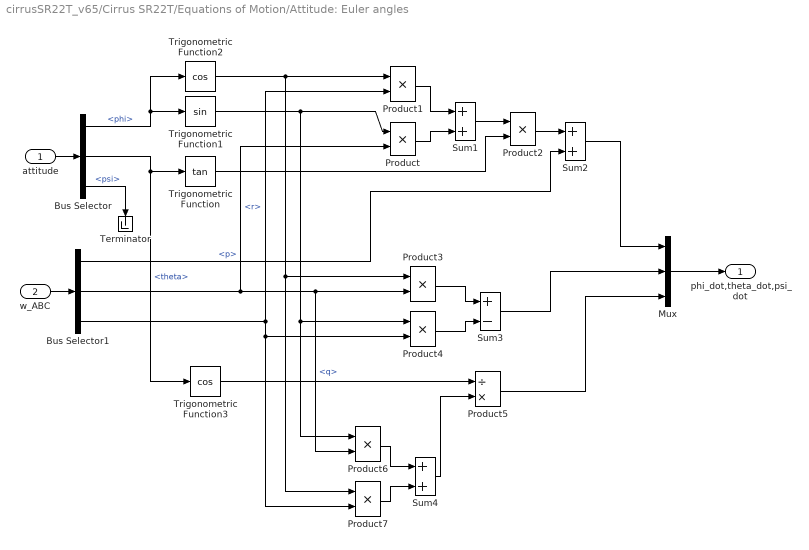
== system cirrusSR22T_v65/Cirrus SR22T/Equations of Motion/Attitude: Euler angles ==
  attitude : Inport
  w_ABC : Inport  Port=2
  Bus Selector : BusSelector  OutputSignals=phi,theta,psi
  Bus Selector1 : BusSelector  OutputSignals=p,q,r
  Mux : Mux  Inputs=3
  Product{,1..4,6..7} (7 alike) : Product  SaturateOnIntegerOverflow=on  OutDataTypeStr=Inherit: Same as first input
  Product5 : Product  Inputs=/*  SaturateOnIntegerOverflow=on  OutDataTypeStr=Inherit: Same as first input
  Sum1 : Sum  SaturateOnIntegerOverflow=on
  Sum2 : Sum  SaturateOnIntegerOverflow=on
  Sum3 : Sum  Inputs=+-  SaturateOnIntegerOverflow=on
  Sum4 : Sum  SaturateOnIntegerOverflow=on
  Terminator : Terminator
  Trigonometric Function : Trigonometry  Operator=tan
  Trigonometric Function1 : Trigonometry
  Trigonometric Function2 : Trigonometry  Operator=cos
  Trigonometric Function3 : Trigonometry  Operator=cos
  phi_dot,theta_dot,psi_dot : Outport
  wires:
  Bus Selector/2 -> Trigonometric Function3/1, Trigonometric Function/1  "<theta>"
  Bus Selector/1 -> Trigonometric Function1/1, Trigonometric Function2/1  "<phi>"
  Trigonometric Function1/1 -> Product/1, Product4/1, Product6/1
  Trigonometric Function2/1 -> Product1/1, Product3/1, Product7/1
  Product1/1 -> Sum1/1
  Product/1 -> Sum1/2
  Sum1/1 -> Product2/1
  Product2/1 -> Sum2/1
  Sum2/1 -> Mux/1
  attitude/1 -> Bus Selector/1
  Bus Selector/3 -> Terminator/1  "<psi>"
  Product3/1 -> Sum3/1
  w_ABC/1 -> Bus Selector1/1
  Product4/1 -> Sum3/2
  Trigonometric Function3/1 -> Product5/1
  Product6/1 -> Sum4/1
  Product7/1 -> Sum4/2
  Sum4/1 -> Product5/2
  Sum3/1 -> Mux/2
  Product5/1 -> Mux/3
  Bus Selector1/1 -> Sum2/2  "<p>"
  Mux/1 -> phi_dot,theta_dot,psi_dot/1
  Bus Selector1/2 -> Product/2, Product3/2, Product6/2  "<q>"
  Bus Selector1/3 -> Product1/2, Product4/2, Product7/2  "<r>"
  Trigonometric Function/1 -> Product2/2

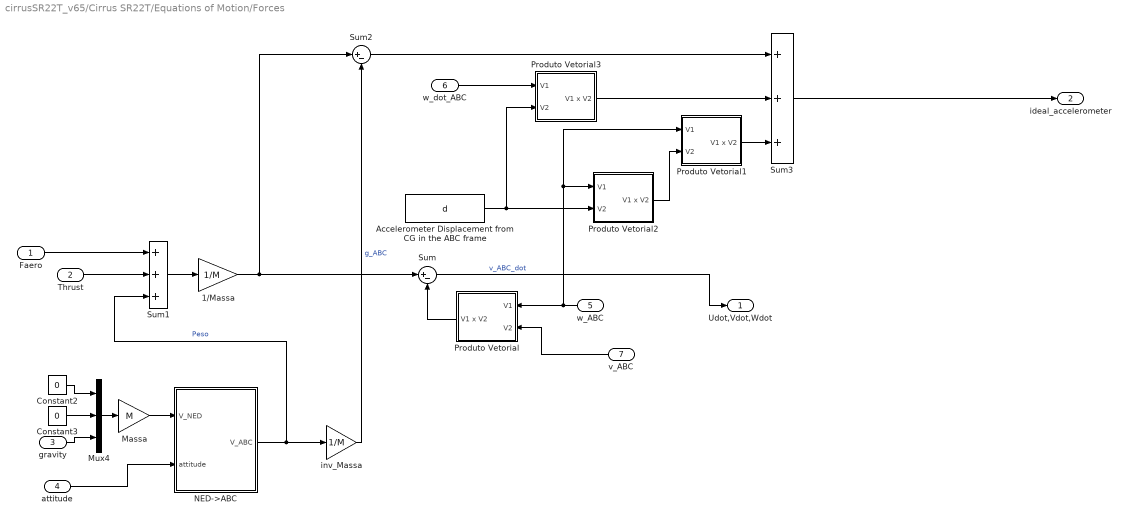
== system cirrusSR22T_v65/Cirrus SR22T/Equations of Motion/Forces ==
  Faero : Inport
  Thrust : Inport  Port=2
  gravity : Inport  Port=3
  attitude : Inport  Port=4
  w_ABC : Inport  Port=5
  w_dot_ABC : Inport  Port=6
  v_ABC : Inport  Port=7
  1/Massa : Gain  Gain=1/M  SaturateOnIntegerOverflow=on  OutDataTypeStr=Inherit: Same as input  ParamDataTypeStr=Inherit: Same as input
  Accelerometer Displacement from CG in the ABC frame : Constant  Value=d
  Constant2 : Constant  Value=0
  Constant3 : Constant  Value=0
  Massa : Gain  Gain=M  SaturateOnIntegerOverflow=on  OutDataTypeStr=Inherit: Same as input  ParamDataTypeStr=Inherit: Same as input
  Mux4 : Mux  Inputs=3
  NED->ABC : Subsystem
  Produto Vetorial : Subsystem
  Produto Vetorial1 : Subsystem
  Produto Vetorial2 : Subsystem
  Produto Vetorial3 : Subsystem
  Sum : Sum  Inputs=|+-  SaturateOnIntegerOverflow=on
  Sum1 : Sum  Inputs=+++  SaturateOnIntegerOverflow=on
  Sum2 : Sum  Inputs=|+-  SaturateOnIntegerOverflow=on
  Sum3 : Sum  Inputs=+++  SaturateOnIntegerOverflow=on
  inv_Massa : Gain  Gain=1/M  SaturateOnIntegerOverflow=on  OutDataTypeStr=Inherit: Same as input  ParamDataTypeStr=Inherit: Same as input
  Udot,Vdot,Wdot : Outport
  ideal_accelerometer : Outport  Port=2
  wires:
  1/Massa/1 -> Sum/1, Sum2/1
  Produto Vetorial/1(V1 x V2) -> Sum/2
  w_ABC/1 -> Produto Vetorial/1(V1), Produto Vetorial2/1(V1), Produto Vetorial1/1(V1)
  v_ABC/1 -> Produto Vetorial/2(V2)
  Sum1/1 -> 1/Massa/1
  Constant2/1 -> Mux4/1
  Constant3/1 -> Mux4/2
  gravity/1 -> Mux4/3
  Mux4/1 -> Massa/1
  Massa/1 -> NED->ABC/1(V_NED)
  attitude/1 -> NED->ABC/2(attitude)
  Faero/1 -> Sum1/1
  Thrust/1 -> Sum1/2
  Sum/1 -> Udot,Vdot,Wdot/1  "v_ABC_dot"
  NED->ABC/1(V_ABC) -> Sum1/3, inv_Massa/1  "Peso"
  inv_Massa/1 -> Sum2/2  "g_ABC"
  Sum2/1 -> Sum3/1
  Sum3/1 -> ideal_accelerometer/1
  Produto Vetorial2/1(V1 x V2) -> Produto Vetorial1/2(V2)
  Accelerometer Displacement from CG in the ABC frame/1 -> Produto Vetorial2/2(V2), Produto Vetorial3/2(V2)
  Produto Vetorial1/1(V1 x V2) -> Sum3/3
  Produto Vetorial3/1(V1 x V2) -> Sum3/2
  w_dot_ABC/1 -> Produto Vetorial3/1(V1)

== system cirrusSR22T_v65/Cirrus SR22T/Equations of Motion/Moments ==
  Maero : Inport
  Faero : Inport  Port=2
  thrust : Inport  Port=3
  w_ABC : Inport  Port=4
  Aerodynamic Forces point of application : Constant  Value=Aero_RP
  C.G. position : Constant  Value=Rcg
  Engine position : Constant  Value=Rengine
  Inertia : Subsystem
  Inverse Inertia Matrix : Subsystem
  Product : Product  Multiplication=Matrix(*)  SaturateOnIntegerOverflow=on  OutDataTypeStr=Inherit: Same as first input
  Product1 : Product  Multiplication=Matrix(*)  SaturateOnIntegerOverflow=on  OutDataTypeStr=Inherit: Same as first input
  Product2 : Product  Multiplication=Matrix(*)  SaturateOnIntegerOverflow=on  OutDataTypeStr=Inherit: Same as first input
  Produto Vetorial1 : Subsystem
  Produto Vetorial2 : Subsystem
  Produto Vetorial3 : Subsystem
  Sum2 : Sum  Inputs=+++  SaturateOnIntegerOverflow=on
  Sum3 : Sum  Inputs=|+-  SaturateOnIntegerOverflow=on
  Sum4 : Sum  Inputs=|-+  SaturateOnIntegerOverflow=on
  Sum5 : Sum  Inputs=|+-  SaturateOnIntegerOverflow=on
  Pdot,Qdot,Rdot : Outport
  wires:
  Inverse Inertia Matrix/1(inv J) -> Product/1, Product2/1
  Sum2/1 -> Product/2
  Product/1 -> Sum3/1
  Inertia/1(J) -> Product1/1
  w_ABC/1 -> Product1/2, Produto Vetorial1/1(V1)
  Product1/1 -> Produto Vetorial1/2(V2)
  Produto Vetorial1/1(V1 x V2) -> Product2/2
  Product2/1 -> Sum3/2
  C.G. position/1 -> Sum4/1, Sum5/2
  Aerodynamic Forces point of application/1 -> Sum4/2
  Engine position/1 -> Sum5/1
  Sum5/1 -> Produto Vetorial2/1(V1)
  Sum4/1 -> Produto Vetorial3/1(V1)
  Faero/1 -> Produto Vetorial3/2(V2)
  Produto Vetorial3/1(V1 x V2) -> Sum2/3
  Produto Vetorial2/1(V1 x V2) -> Sum2/2
  thrust/1 -> Produto Vetorial2/2(V2)
  Sum3/1 -> Pdot,Qdot,Rdot/1
  Maero/1 -> Sum2/1

== system cirrusSR22T_v65/Cirrus SR22T/Equations of Motion/mod pi1 ==
  u : Inport
  Abs : Abs
  Constant : Constant  Value=pi
  Fcn : Fcn  Expr=u/pi
  Fcn1 : Fcn  Expr=u*pi
  Gain : Gain  Gain=1/2  SaturateOnIntegerOverflow=on  OutDataTypeStr=Inherit: Same as input  ParamDataTypeStr=Inherit: Same as input
  Gain1 : Gain  Gain=2  SaturateOnIntegerOverflow=on  OutDataTypeStr=Inherit: Same as input  ParamDataTypeStr=Inherit: Same as input
  Product : Product  SaturateOnIntegerOverflow=on  OutDataTypeStr=Inherit: Same as first input
  Rounding Function : Rounding  Operator=fix
  Rounding Function1 : Rounding  Operator=fix
  Sign : Signum
  Sum : Sum  Inputs=|-+  SaturateOnIntegerOverflow=on
  Sum1 : Sum  Inputs=-+|  SaturateOnIntegerOverflow=on
  Sum2 : Sum  Inputs=+-|  SaturateOnIntegerOverflow=on
  Switch1 : Switch  Threshold=0.5  InputSameDT=off
  y : Outport
  wires:
  u/1 -> Abs/1, Sign/1
  Fcn/1 -> Rounding Function/1
  Rounding Function/1 -> Fcn1/1, Gain/1, Sum2/1
  Fcn1/1 -> Sum/1
  Abs/1 -> Fcn/1, Sum/2
  Sign/1 -> Product/2
  Product/1 -> y/1
  Sum/1 -> Sum1/2, Switch1/3
  Constant/1 -> Sum1/1
  Sum1/1 -> Switch1/1
  Switch1/1 -> Product/1
  Gain/1 -> Rounding Function1/1
  Rounding Function1/1 -> Gain1/1
  Gain1/1 -> Sum2/2
  Sum2/1 -> Switch1/2

== system cirrusSR22T_v65/Cirrus SR22T/Equations of Motion/mod pi2 ==
  u : Inport
  Abs : Abs
  Constant : Constant  Value=pi
  Fcn : Fcn  Expr=u/pi
  Fcn1 : Fcn  Expr=u*pi
  Gain : Gain  Gain=1/2  SaturateOnIntegerOverflow=on  OutDataTypeStr=Inherit: Same as input  ParamDataTypeStr=Inherit: Same as input
  Gain1 : Gain  Gain=2  SaturateOnIntegerOverflow=on  OutDataTypeStr=Inherit: Same as input  ParamDataTypeStr=Inherit: Same as input
  Product : Product  SaturateOnIntegerOverflow=on  OutDataTypeStr=Inherit: Same as first input
  Rounding Function : Rounding  Operator=fix
  Rounding Function1 : Rounding  Operator=fix
  Sign : Signum
  Sum : Sum  Inputs=|-+  SaturateOnIntegerOverflow=on
  Sum1 : Sum  Inputs=-+|  SaturateOnIntegerOverflow=on
  Sum2 : Sum  Inputs=+-|  SaturateOnIntegerOverflow=on
  Switch1 : Switch  Threshold=0.5  InputSameDT=off
  y : Outport
  wires:
  u/1 -> Abs/1, Sign/1
  Fcn/1 -> Rounding Function/1
  Rounding Function/1 -> Fcn1/1, Gain/1, Sum2/1
  Fcn1/1 -> Sum/1
  Abs/1 -> Fcn/1, Sum/2
  Sign/1 -> Product/2
  Product/1 -> y/1
  Sum/1 -> Sum1/2, Switch1/3
  Constant/1 -> Sum1/1
  Sum1/1 -> Switch1/1
  Switch1/1 -> Product/1
  Gain/1 -> Rounding Function1/1
  Rounding Function1/1 -> Gain1/1
  Gain1/1 -> Sum2/2
  Sum2/1 -> Switch1/2

== system cirrusSR22T_v65/Cirrus SR22T/Equations of Motion/mod pi3 ==
  u : Inport
  Abs : Abs
  Constant : Constant  Value=pi
  Fcn : Fcn  Expr=u/pi
  Fcn1 : Fcn  Expr=u*pi
  Gain : Gain  Gain=1/2  SaturateOnIntegerOverflow=on  OutDataTypeStr=Inherit: Same as input  ParamDataTypeStr=Inherit: Same as input
  Gain1 : Gain  Gain=2  SaturateOnIntegerOverflow=on  OutDataTypeStr=Inherit: Same as input  ParamDataTypeStr=Inherit: Same as input
  Product : Product  SaturateOnIntegerOverflow=on  OutDataTypeStr=Inherit: Same as first input
  Rounding Function : Rounding  Operator=fix
  Rounding Function1 : Rounding  Operator=fix
  Sign : Signum
  Sum : Sum  Inputs=|-+  SaturateOnIntegerOverflow=on
  Sum1 : Sum  Inputs=-+|  SaturateOnIntegerOverflow=on
  Sum2 : Sum  Inputs=+-|  SaturateOnIntegerOverflow=on
  Switch1 : Switch  Threshold=0.5  InputSameDT=off
  y : Outport
  wires:
  u/1 -> Abs/1, Sign/1
  Fcn/1 -> Rounding Function/1
  Rounding Function/1 -> Fcn1/1, Gain/1, Sum2/1
  Fcn1/1 -> Sum/1
  Abs/1 -> Fcn/1, Sum/2
  Sign/1 -> Product/2
  Product/1 -> y/1
  Sum/1 -> Sum1/2, Switch1/3
  Constant/1 -> Sum1/1
  Sum1/1 -> Switch1/1
  Switch1/1 -> Product/1
  Gain/1 -> Rounding Function1/1
  Rounding Function1/1 -> Gain1/1
  Gain1/1 -> Sum2/2
  Sum2/1 -> Switch1/2

== system cirrusSR22T_v65/Cirrus SR22T/Equations of Motion/position ==
  V_ABC : Inport
  attitude : Inport  Port=2
  ABC->NED : Subsystem
  Constant : Constant  Value=0  VectorParams1D=off
  Constant1 : Constant  Value=isTrimming  VectorParams1D=off
  Demux1 : Demux  Outputs=3
      settings: DisplayOption=none
  Gain : Gain  Gain=-1  SaturateOnIntegerOverflow=on  OutDataTypeStr=Inherit: Same as input  ParamDataTypeStr=Inherit: Same as input
  Mux : Mux  Inputs=3
  Switch : Switch  Threshold=0.5  InputSameDT=off
  Switch1 : Switch  Threshold=0.5  InputSameDT=off
  V_NED : Outport
  wires:
  ABC->NED/1(V_NED) -> Demux1/1
  V_ABC/1 -> ABC->NED/1(V_ABC)
  attitude/1 -> ABC->NED/2(attitude)
  Demux1/3 -> Gain/1  "-h"
  Gain/1 -> Mux/3
  Mux/1 -> V_NED/1
  Switch/1 -> Mux/1
  Demux1/1 -> Switch/3  "V_N"
  Switch1/1 -> Mux/2
  Demux1/2 -> Switch1/3  "V_E"
  Constant/1 -> Switch/1, Switch1/1
  Constant1/1 -> Switch/2, Switch1/2

== system cirrusSR22T_v65/Cirrus SR22T/Aerodinamica/Forcas Aerodinamicas/Coef. Arrasto ==
  alpha : Inport
  beta : Inport  Port=2
  elevator : Inport  Port=3
  C_L : Inport  Port=4
  Mach : Inport  Port=5
  Abs : Abs  SaturateOnIntegerOverflow=off
  CD_alpha : Lookup  InputValues=CD_alpha(:,1);  Table=CD_alpha(:,2);  LookUpMeth=Interpolation-Use End Values
  CD_beta : Lookup  InputValues=CD_beta(:,1);  Table=CD_beta(:,2);  LookUpMeth=Interpolation-Use End Values
  CD_mach : Lookup  InputValues=CD_mach(:,1);  Table=CD_mach(:,2);  LookUpMeth=Interpolation-Use End Values
  Constant : Constant  Value=0
  Gain : Gain  Gain=CD_elev
  Gain1 : Gain  Gain=CD_ind
  Norm : Gain  Gain=1/0.35
  Square : Math  Operator=square
  Sum : Sum  Inputs=++++++  SaturateOnIntegerOverflow=on
  C_D : Outport
  wires:
  alpha/1 -> CD_alpha/1
  Constant/1 -> Sum/1
  CD_alpha/1 -> Sum/2  "CD_alpha_sim"
  CD_beta/1 -> Sum/3  "CD_beta_sim"
  beta/1 -> CD_beta/1
  Sum/1 -> C_D/1  "C_D_sim"
  elevator/1 -> Abs/1
  Abs/1 -> Gain/1
  C_L/1 -> Square/1
  Square/1 -> Gain1/1
  Gain1/1 -> Sum/5  "CD_ind_sim"
  Mach/1 -> CD_mach/1
  CD_mach/1 -> Sum/6  "CD_mach_sim"
  Gain/1 -> Norm/1
  Norm/1 -> Sum/4  "CD_elev_sim"
